simulink model "ds_pose_test"  (R2019a)
settings: Solver=ode14x  StartTime=0  StopTime=0.001  FixedStep=.00001  RelTol=1e-3  EnableMultiTasking=on
model workspace (MAT data in the model file):
  Ankle_L_D = 0.125126243033
  Ankle_L_S = 0.0328154604487
  Ankle_R_D = 0.245807097642
  Ankle_R_S = 0.682954357178
  BeginTimePlantModel = 0.0498
  F_C = 0.06105
  F_H = 0.07
  F_I = 0.00125071180063
  F_L = 0.185
  F_M = 1.13129
  F_W = 0.1
  GRF_HD = 941.037069119
  GRF_HS = 1691.11560066
  GRF_VD = 12300.8672242
  GRF_VS = 71710.3574634
  HAT_I = 3.41998320224
  HAT_L = 0.51264
  HAT_M = 52.89756
  HAT_a = 0.2
  HAT_b = 0.11
  Hip_L_D = 0.0332143791481
  Hip_L_S = 0.0516603438036
  Hip_R_D = 0.145088103411
  Hip_R_S = 0.15911410017
  Knee_L_D = 0.0558982452805
  Knee_L_S = 0.00250387295429
  Knee_R_D = 0.0619293882143
  Knee_R_S = 0.0623339259595
  M : struct (value not decoded)
  S_I = 0.0556212184297
  S_L = 0.41
  S_M = 3.62793
  S_R1 = 0.035
  S_R2 = 0.0716197243914
  T_I = 0.63371745
  T_L = 0.6
  T_M = 7.802
  T_R1 = 0.0716197243914
  T_R2 = 0.105042262441
  bodymass = 78.02
  p_stance_ankle = 14.9539905036
  p_stance_hip = -24.9413676415
  p_stance_knee = -2.50807459996
  p_swing_ankle = 4.11757124464
  p_swing_hip = 18.3000604838
  p_swing_knee = -3.41741510381
  polyfit_stance_ankle = [-863347.977095 222377.922877 -7468.35453889 -9.40558010807 -153.06789694]
  polyfit_stance_hip = [-279786636.688 114363391.625 -15725654.0525 856134.662579 -22930.0516399 481.110496147 63.2694363354]
  polyfit_stance_knee = [-122862314.114 52903969.6705 -7988612.27678 487806.049871 -8969.32141641 330.337585729 -54.0526736443]
  polyfit_swing_ankle = [49510154320.8 -30205907167.6 7312588550.85 -888915044.437 56385922.5861 -1769074.37171 25613.4020917 -113.306543933 -1.03720591697]
  polyfit_swing_hip = [538683495113 -366532634246 101719653645 -14750073882.9 1184454520.37 -50949861.1242 1019832.60417 -6310.84925925 -38.0907282261]
  polyfit_swing_knee = [352478408737 -233011269241 62650744932.5 -8775138187.04 678489689.503 -28060179.8998 545151.783137 -3282.03325692 -26.455631467]
  stance_hip_D = -0.1
  stance_hip_I = 0
  stance_hip_P = -1
  swing_hip_D = -0.1
  swing_hip_I = 0
  swing_hip_P = -1
  u_stance_ankle = [69.4103486139 -2.96655029606 -0.484600956449 15.837035075 -30.2582315444 74.2176519508]
  u_stance_knee = [13.7314398955 -29.9969611778 1.73615680112 0.18917262326 19.1195166289 -5.6755240825]
  u_swing_ankle = [1.12328276614 1.37618839903 0.187919802027 3.02355316687 -2.87615035677 -3.05964445898]
  u_swing_knee = [0.261233056105 2.98474073296 -1.89258958543 4.37484849204 4.7809069003 3.51361766866]
  w_stance_ankle = 38.5856494503
  w_stance_hip = -48.9218873275
  w_stance_knee = 204.10219458
  w_swing_ankle = -56.5478745686
  w_swing_hip = 64.9583214539
  w_swing_knee = 388.822549535
  x_planar_p = 0
  x_planar_v = 0
  y_planar_p = 0
  y_planar_v = 0
  yout = [8.16988597066 8.1627557225 8.15559878707 8.14841513681 8.14120474348 8.13396757813 8.12670361115 8.11941281227 8.1120951506 8.10475059463 8.09737911226 8.08998067083 ... (8000 elements, 1000x8)]
  z_planar_p = -10.3139246991
  z_planar_w = -47.4942945829
values from neighbouring files (symbols this model uses):
  N = 3    [lagdmodel.m]
symbols that are objects in the model workspace (value not decoded): M
undefined symbols (not defined in the file or in its folder): X, Y, Z
libraries: nesl_utility x87, sm_lib x51, fl_lib x24, fl_ps_legacy_lib x16, simulink x4
(part 9 of 9)

== system ds_pose_test/Foot_R/Heel_GRF/Subsystem ==
  Constant : Constant  Value=0
  Constant1 : Constant  Value=0
  Damping : Switch
  Gain : Gain  Gain=-GRF_VS
  Gain1 : Gain  Gain=-GRF_VD
  PS-Simulink Converter : nesl_utility/PS-Simulink Converter  PhysicalDomain=network_engine_domain  SubClassName=ps_output  LeftPortType=input  RightPortType=output  PseudoPeriodic=off  Frequencies=[]  Unit=1  AffineConversion=off
  PS-Simulink Converter1 : nesl_utility/PS-Simulink Converter  PhysicalDomain=network_engine_domain  SubClassName=ps_output  LeftPortType=input  RightPortType=output  PseudoPeriodic=off  Frequencies=[]  Unit=1  AffineConversion=off
  Scope : Scope
  Scope1 : Scope
  Scope2 : Scope
  Simulink-PS Converter : nesl_utility/Simulink-PS Converter  PhysicalDomain=network_engine_domain  SubClassName=ps_input  LeftPortType=input  RightPortType=output  PseudoPeriodic=off  Frequencies=[]  NoiseDistribution=none  NoiseParameters=[]  Unit=1  AffineConversion=off  FilteringAndDerivatives=zero  SimscapeFilterOrder=1  InputFilterTimeConstant=.001  UdotUserProvided=[]
  Spring : Switch
  Sum : Sum  Inputs=|++
  Vertical Force : PMIOPort  Side=Right
  Vertical Position : PMIOPort  Port=2  Side=Left
  Vertical Velocity : PMIOPort  Port=3  Side=Left
  wires:
  Damping/1 -> Sum/2
  Spring/1 -> Sum/1
  PS-Simulink Converter1/1 -> Scope1/1, Gain1/1
  Gain1/1 -> Damping/3
  Constant1/1 -> Damping/1
  Constant/1 -> Spring/1
  Gain/1 -> Spring/3
  PS-Simulink Converter/1 -> Scope/1, Gain/1, Damping/2, Spring/2
  Sum/1 -> Scope2/1, Simulink-PS Converter/1
  connections:
  Vertical Position/RConn1 -- PS-Simulink Converter/LConn1
  Vertical Velocity/RConn1 -- PS-Simulink Converter1/LConn1
  Simulink-PS Converter/RConn1 -- Vertical Force/RConn1

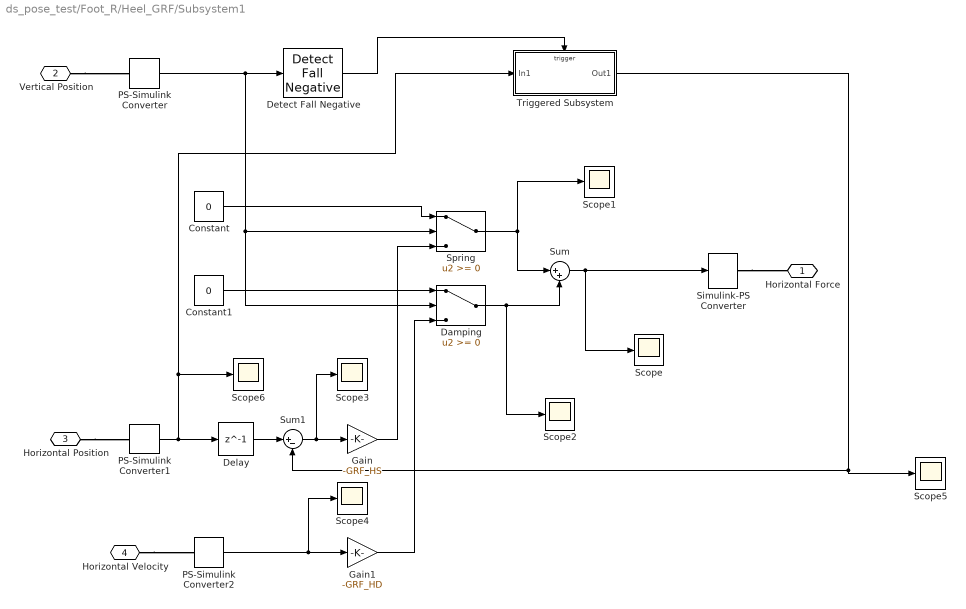
== system ds_pose_test/Foot_R/Heel_GRF/Subsystem1 ==
  Constant : Constant  Value=0
  Constant1 : Constant  Value=0
  Damping : Switch
  Delay : Delay  DelayLength=1  InitialCondition=0
  Detect Fall Negative : simulink/Logic and Bit Operations/Detect Fall Negative  vinit=0  OutDataTypeStr=boolean
      settings: SourceProductName=Simulink  SourceProductBaseCode=SL
  Gain : Gain  Gain=-GRF_HS
  Gain1 : Gain  Gain=-GRF_HD
  PS-Simulink Converter : nesl_utility/PS-Simulink Converter  PhysicalDomain=network_engine_domain  SubClassName=ps_output  LeftPortType=input  RightPortType=output  PseudoPeriodic=off  Frequencies=[]  Unit=1  AffineConversion=off
  PS-Simulink Converter1 : nesl_utility/PS-Simulink Converter  PhysicalDomain=network_engine_domain  SubClassName=ps_output  LeftPortType=input  RightPortType=output  PseudoPeriodic=off  Frequencies=[]  Unit=1  AffineConversion=off
  PS-Simulink Converter2 : nesl_utility/PS-Simulink Converter  PhysicalDomain=network_engine_domain  SubClassName=ps_output  LeftPortType=input  RightPortType=output  PseudoPeriodic=off  Frequencies=[]  Unit=1  AffineConversion=off
  Scope{,1..6} (7 alike) : Scope
  Simulink-PS Converter : nesl_utility/Simulink-PS Converter  PhysicalDomain=network_engine_domain  SubClassName=ps_input  LeftPortType=input  RightPortType=output  PseudoPeriodic=off  Frequencies=[]  NoiseDistribution=none  NoiseParameters=[]  Unit=1  AffineConversion=off  FilteringAndDerivatives=zero  SimscapeFilterOrder=1  InputFilterTimeConstant=.001  UdotUserProvided=[]
  Spring : Switch
  Sum : Sum  Inputs=|++
  Sum1 : Sum  Inputs=|+-
  Triggered Subsystem : Subsystem  TreatAsAtomicUnit=on
  Horizontal Force : PMIOPort  Side=Right
  Vertical Position : PMIOPort  Port=2  Side=Left
  Horizontal Position : PMIOPort  Port=3  Side=Left
  Horizontal Velocity : PMIOPort  Port=4  Side=Left
  wires:
  Spring/1 -> Scope1/1, Sum/1
  Damping/1 -> Scope2/1, Sum/2
  PS-Simulink Converter2/1 -> Scope4/1, Gain1/1
  PS-Simulink Converter1/1 -> Triggered Subsystem/1(In1), Scope6/1, Delay/1
  Sum1/1 -> Scope3/1, Gain/1
  Sum/1 -> Simulink-PS Converter/1, Scope/1
  PS-Simulink Converter/1 -> Detect Fall Negative/1, Spring/2, Damping/2
  Detect Fall Negative/1 -> Triggered Subsystem/Trigger
  Triggered Subsystem/1(Out1) -> Sum1/2, Scope5/1
  Delay/1 -> Sum1/1
  Constant/1 -> Spring/1
  Constant1/1 -> Damping/1
  Gain/1 -> Spring/3
  Gain1/1 -> Damping/3
  connections:
  Vertical Position/RConn1 -- PS-Simulink Converter/LConn1
  Horizontal Position/RConn1 -- PS-Simulink Converter1/LConn1
  Horizontal Velocity/RConn1 -- PS-Simulink Converter2/LConn1
  Simulink-PS Converter/RConn1 -- Horizontal Force/RConn1

== system ds_pose_test/Foot_R/Toe_GRF /Subsystem ==
  Constant : Constant  Value=0
  Constant1 : Constant  Value=0
  Damping : Switch
  Gain : Gain  Gain=-GRF_VS
  Gain1 : Gain  Gain=-GRF_VD
  PS-Simulink Converter : nesl_utility/PS-Simulink Converter  PhysicalDomain=network_engine_domain  SubClassName=ps_output  LeftPortType=input  RightPortType=output  PseudoPeriodic=off  Frequencies=[]  Unit=1  AffineConversion=off
  PS-Simulink Converter1 : nesl_utility/PS-Simulink Converter  PhysicalDomain=network_engine_domain  SubClassName=ps_output  LeftPortType=input  RightPortType=output  PseudoPeriodic=off  Frequencies=[]  Unit=1  AffineConversion=off
  Scope : Scope
  Scope1 : Scope
  Scope2 : Scope
  Simulink-PS Converter : nesl_utility/Simulink-PS Converter  PhysicalDomain=network_engine_domain  SubClassName=ps_input  LeftPortType=input  RightPortType=output  PseudoPeriodic=off  Frequencies=[]  NoiseDistribution=none  NoiseParameters=[]  Unit=1  AffineConversion=off  FilteringAndDerivatives=zero  SimscapeFilterOrder=1  InputFilterTimeConstant=.001  UdotUserProvided=[]
  Spring : Switch
  Sum : Sum  Inputs=|++
  Vertical Force : PMIOPort  Side=Right
  Vertical Position : PMIOPort  Port=2  Side=Left
  Vertical Velocity : PMIOPort  Port=3  Side=Left
  wires:
  Damping/1 -> Sum/2
  Spring/1 -> Sum/1
  PS-Simulink Converter1/1 -> Scope1/1, Gain1/1
  Gain1/1 -> Damping/3
  Constant1/1 -> Damping/1
  Constant/1 -> Spring/1
  Gain/1 -> Spring/3
  PS-Simulink Converter/1 -> Scope/1, Gain/1, Damping/2, Spring/2
  Sum/1 -> Scope2/1, Simulink-PS Converter/1
  connections:
  Vertical Position/RConn1 -- PS-Simulink Converter/LConn1
  Vertical Velocity/RConn1 -- PS-Simulink Converter1/LConn1
  Simulink-PS Converter/RConn1 -- Vertical Force/RConn1

== system ds_pose_test/Foot_R/Toe_GRF /Subsystem1 ==
  Constant : Constant  Value=0
  Constant1 : Constant  Value=0
  Damping : Switch
  Delay : Delay  DelayLength=1  InitialCondition=0
  Detect Fall Negative : simulink/Logic and Bit Operations/Detect Fall Negative  vinit=0  OutDataTypeStr=boolean
      settings: SourceProductName=Simulink  SourceProductBaseCode=SL
  Gain : Gain  Gain=-GRF_HS
  Gain1 : Gain  Gain=-GRF_HD
  PS-Simulink Converter : nesl_utility/PS-Simulink Converter  PhysicalDomain=network_engine_domain  SubClassName=ps_output  LeftPortType=input  RightPortType=output  PseudoPeriodic=off  Frequencies=[]  Unit=1  AffineConversion=off
  PS-Simulink Converter1 : nesl_utility/PS-Simulink Converter  PhysicalDomain=network_engine_domain  SubClassName=ps_output  LeftPortType=input  RightPortType=output  PseudoPeriodic=off  Frequencies=[]  Unit=1  AffineConversion=off
  PS-Simulink Converter2 : nesl_utility/PS-Simulink Converter  PhysicalDomain=network_engine_domain  SubClassName=ps_output  LeftPortType=input  RightPortType=output  PseudoPeriodic=off  Frequencies=[]  Unit=1  AffineConversion=off
  Scope{,1..2,4} (4 alike) : Scope
  Simulink-PS Converter : nesl_utility/Simulink-PS Converter  PhysicalDomain=network_engine_domain  SubClassName=ps_input  LeftPortType=input  RightPortType=output  PseudoPeriodic=off  Frequencies=[]  NoiseDistribution=none  NoiseParameters=[]  Unit=1  AffineConversion=off  FilteringAndDerivatives=zero  SimscapeFilterOrder=1  InputFilterTimeConstant=.001  UdotUserProvided=[]
  Spring : Switch
  Sum : Sum  Inputs=|++
  Sum1 : Sum  Inputs=|+-
  Triggered Subsystem : Subsystem  TreatAsAtomicUnit=on
  Horizontal Force : PMIOPort  Side=Right
  Vertical Position : PMIOPort  Port=2  Side=Left
  Horizontal Position : PMIOPort  Port=3  Side=Left
  Horizontal Velocity : PMIOPort  Port=4  Side=Left
  wires:
  Spring/1 -> Scope1/1, Sum/1
  Damping/1 -> Scope2/1, Sum/2
  PS-Simulink Converter2/1 -> Scope4/1, Gain1/1
  PS-Simulink Converter1/1 -> Triggered Subsystem/1(In1), Delay/1
  Sum1/1 -> Gain/1
  Sum/1 -> Simulink-PS Converter/1, Scope/1
  Gain/1 -> Spring/3
  Gain1/1 -> Damping/3
  Constant/1 -> Spring/1
  Constant1/1 -> Damping/1
  PS-Simulink Converter/1 -> Damping/2, Spring/2, Detect Fall Negative/1
  Detect Fall Negative/1 -> Triggered Subsystem/Trigger
  Triggered Subsystem/1(Out1) -> Sum1/2
  Delay/1 -> Sum1/1
  connections:
  Vertical Position/RConn1 -- PS-Simulink Converter/LConn1
  Horizontal Position/RConn1 -- PS-Simulink Converter1/LConn1
  Horizontal Velocity/RConn1 -- PS-Simulink Converter2/LConn1
  Simulink-PS Converter/RConn1 -- Horizontal Force/RConn1

== system ds_pose_test/Hip_L_PID_Control/Hip_L_Actuation1/Hard_Stop_Hip_L ==
  Mechanical Rotational Reference : fl_lib/Mechanical/Rotational Elements/Mechanical Rotational Reference
  Rotational Simscape Intf (Library Block) : Subsystem
  Rotational Hard Stop : fl_lib/Mechanical/Rotational Elements/Rotational Hard Stop  upper_bnd=upper_bound rad  lower_bnd=lower_bound rad  stiff_up=contact_stiffness N*m/rad  stiff_low=contact_stiffness N*m/rad  D_up=contact_damping N*m/(rad/s)  D_low=contact_damping N*m/(rad/s)  model=3  transition=0.001 rad  w_specify=off  w_priority=None  w=0 rad/s  w_nominal_specify=off  w_nominal_unit=rad/s  w_nominal_value=1  t_specify=off  t_priority=None  t=0 N*m  t_nominal_specify=off  t_nominal_unit=N*m  t_nominal_value=1  phi_specify=on  phi_priority=High  phi=initial_angular_position rad  phi_nominal_specify=off  phi_nominal_unit=rad  phi_nominal_value=1
      settings: SourceProductName=Simscape  SourceProductBaseCode=SS
  T : PMIOPort  Side=Right
  w : PMIOPort  Port=2  Side=Left
  connections:
  Rotational Simscape Intf (Library Block)/LConn2 -- Rotational Hard Stop/LConn1 -- Mechanical Rotational Reference/LConn1
  Rotational Hard Stop/RConn1 -- Rotational Simscape Intf (Library Block)/RConn2
  w/RConn1 -- Rotational Simscape Intf (Library Block)/LConn1
  Rotational Simscape Intf (Library Block)/RConn1 -- T/RConn1

== system ds_pose_test/Hip_R_PID_Control1/Hip_R_Actuation1/Hard_Stop_Hip_L ==
  Mechanical Rotational Reference : fl_lib/Mechanical/Rotational Elements/Mechanical Rotational Reference
  Rotational Simscape Intf (Library Block) : Subsystem
  Rotational Hard Stop : fl_lib/Mechanical/Rotational Elements/Rotational Hard Stop  upper_bnd=upper_bound rad  lower_bnd=lower_bound rad  stiff_up=contact_stiffness N*m/rad  stiff_low=contact_stiffness N*m/rad  D_up=contact_damping N*m/(rad/s)  D_low=contact_damping N*m/(rad/s)  model=3  transition=0.001 rad  w_specify=off  w_priority=None  w=0 rad/s  w_nominal_specify=off  w_nominal_unit=rad/s  w_nominal_value=1  t_specify=off  t_priority=None  t=0 N*m  t_nominal_specify=off  t_nominal_unit=N*m  t_nominal_value=1  phi_specify=on  phi_priority=High  phi=initial_angular_position rad  phi_nominal_specify=off  phi_nominal_unit=rad  phi_nominal_value=1
      settings: SourceProductName=Simscape  SourceProductBaseCode=SS
  T : PMIOPort  Side=Right
  w : PMIOPort  Port=2  Side=Left
  connections:
  Rotational Simscape Intf (Library Block)/LConn2 -- Rotational Hard Stop/LConn1 -- Mechanical Rotational Reference/LConn1
  Rotational Hard Stop/RConn1 -- Rotational Simscape Intf (Library Block)/RConn2
  w/RConn1 -- Rotational Simscape Intf (Library Block)/LConn1
  Rotational Simscape Intf (Library Block)/RConn1 -- T/RConn1

== system ds_pose_test/Knee_L_Actuation/Hard_Stop_Knee_L/Rotational Simscape Intf (Library Block) ==
  Ideal Angular Velocity Source : fl_lib/Mechanical/Mechanical Sources/Ideal Angular Velocity Source
  Ideal Torque Sensor : fl_lib/Mechanical/Mechanical Sensors/Ideal Torque Sensor
  w : PMIOPort  Side=Left
  T : PMIOPort  Port=2  Side=Right
  R : PMIOPort  Port=3  Side=Left
  C : PMIOPort  Port=4  Side=Right
  connections:
  Ideal Torque Sensor/RConn1 -- C/RConn1
  R/RConn1 -- Ideal Angular Velocity Source/LConn1
  Ideal Torque Sensor/LConn1 -- Ideal Angular Velocity Source/RConn2
  T/RConn1 -- Ideal Torque Sensor/RConn2
  w/RConn1 -- Ideal Angular Velocity Source/RConn1

== system ds_pose_test/Knee_R_Actuation/Hard_Stop_Knee_L1/Rotational Simscape Intf (Library Block) ==
  Ideal Angular Velocity Source : fl_lib/Mechanical/Mechanical Sources/Ideal Angular Velocity Source
  Ideal Torque Sensor : fl_lib/Mechanical/Mechanical Sensors/Ideal Torque Sensor
  w : PMIOPort  Side=Left
  T : PMIOPort  Port=2  Side=Right
  R : PMIOPort  Port=3  Side=Left
  C : PMIOPort  Port=4  Side=Right
  connections:
  Ideal Torque Sensor/RConn1 -- C/RConn1
  R/RConn1 -- Ideal Angular Velocity Source/LConn1
  Ideal Torque Sensor/LConn1 -- Ideal Angular Velocity Source/RConn2
  T/RConn1 -- Ideal Torque Sensor/RConn2
  w/RConn1 -- Ideal Angular Velocity Source/RConn1

== system ds_pose_test/Foot_L/Heel_GRF/Subsystem1/Triggered Subsystem ==
  In1 : Inport
  Trigger : TriggerPort  TriggerType=falling  VariantControl=Variant
  Out1 : Outport
  wires:
  In1/1 -> Out1/1

== system ds_pose_test/Foot_L/Toe_GRF/Subsystem1/Triggered Subsystem ==
  In1 : Inport
  Trigger : TriggerPort  TriggerType=falling  VariantControl=Variant
  Out1 : Outport
  wires:
  In1/1 -> Out1/1

== system ds_pose_test/Foot_R/Heel_GRF/Subsystem1/Triggered Subsystem ==
  In1 : Inport
  Trigger : TriggerPort  TriggerType=falling  VariantControl=Variant
  Out1 : Outport
  wires:
  In1/1 -> Out1/1

== system ds_pose_test/Foot_R/Toe_GRF /Subsystem1/Triggered Subsystem ==
  In1 : Inport
  Trigger : TriggerPort  TriggerType=falling  VariantControl=Variant
  Out1 : Outport
  wires:
  In1/1 -> Out1/1

== system ds_pose_test/Hip_L_PID_Control/Hip_L_Actuation1/Hard_Stop_Hip_L/Rotational Simscape Intf (Library Block) ==
  Ideal Angular Velocity Source : fl_lib/Mechanical/Mechanical Sources/Ideal Angular Velocity Source
  Ideal Torque Sensor : fl_lib/Mechanical/Mechanical Sensors/Ideal Torque Sensor
  w : PMIOPort  Side=Left
  T : PMIOPort  Port=2  Side=Right
  R : PMIOPort  Port=3  Side=Left
  C : PMIOPort  Port=4  Side=Right
  connections:
  w/RConn1 -- Ideal Angular Velocity Source/RConn1
  T/RConn1 -- Ideal Torque Sensor/RConn2
  Ideal Torque Sensor/LConn1 -- Ideal Angular Velocity Source/RConn2
  R/RConn1 -- Ideal Angular Velocity Source/LConn1
  Ideal Torque Sensor/RConn1 -- C/RConn1

== system ds_pose_test/Hip_R_PID_Control1/Hip_R_Actuation1/Hard_Stop_Hip_L/Rotational Simscape Intf (Library Block) ==
  Ideal Angular Velocity Source : fl_lib/Mechanical/Mechanical Sources/Ideal Angular Velocity Source
  Ideal Torque Sensor : fl_lib/Mechanical/Mechanical Sensors/Ideal Torque Sensor
  w : PMIOPort  Side=Left
  T : PMIOPort  Port=2  Side=Right
  R : PMIOPort  Port=3  Side=Left
  C : PMIOPort  Port=4  Side=Right
  connections:
  w/RConn1 -- Ideal Angular Velocity Source/RConn1
  T/RConn1 -- Ideal Torque Sensor/RConn2
  Ideal Torque Sensor/LConn1 -- Ideal Angular Velocity Source/RConn2
  R/RConn1 -- Ideal Angular Velocity Source/LConn1
  Ideal Torque Sensor/RConn1 -- C/RConn1
